simulink model "adcs_sim"  (R2026a)
settings: Solver=ode4  StopTime=t_end  FixedStep=dt
values from neighbouring files (symbols this model uses):
  ephem_moon = [ephem_raw.moon_x, ephem_raw.moon_y, ephem_raw.moon_z]    [init_adcs_params.m]
  ephem_sun = [ephem_raw.sun_x,  ephem_raw.sun_y,  ephem_raw.sun_z]    [init_adcs_params.m]
  ephem_t_sec = seconds(ephem_dt - ephem_epoch)    [init_adcs_params.m]
  epoch_jd = 2461083.5    [init_adcs_params.m]
  h_W0 = [0; 0; 0; 0]    [init_adcs_params.m]
  J = diag([Jx, Jy, Jz])    [Simulator.m]    (also in init_adcs_params.m = diag((mass_sc / 12) * [      sc_dim_y^2 + sc_dim_z^2,      s; summarize_adcs_simulation.m = evalin('base', 'J'))
  omega0 = [0.01; 0.02; 0.0]    [Simulator.m]    (also in init_adcs_params.m = [0.01; -0.005; 0.02]; summarize_adcs_simulation.m = evalin('base', 'omega0'))
  q0 = [1; 0; 0; 0]    [init_adcs_params.m]    (also in launch_adcs_gui.m = q0 / q_norm; summarize_adcs_simulation.m = normalize_quaternion(evalin('base', 'q0')))
settings Model: Creator=akshu  LastModifiedBy=akshu

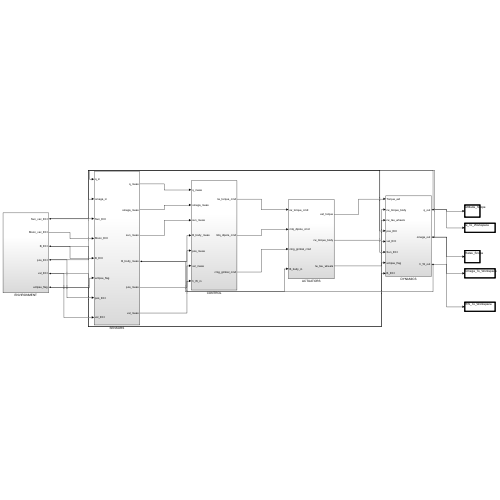
[thumbnail: Simulink's stored preview of the top-level diagram]
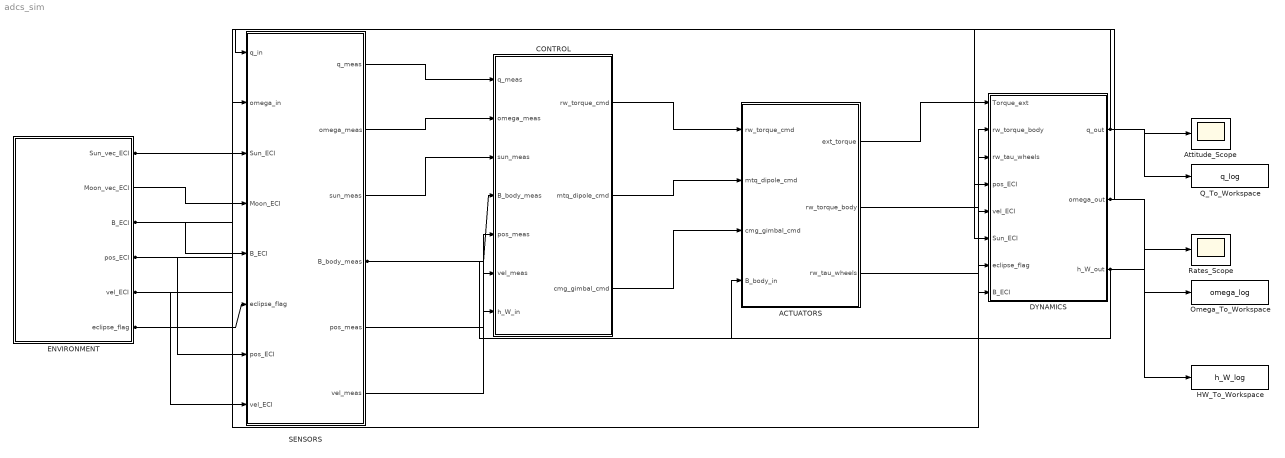
== system adcs_sim ==
  ACTUATORS : Subsystem
  Attitude_Scope : Scope
  CONTROL : Subsystem
  DYNAMICS : Subsystem
  ENVIRONMENT : Subsystem
  HW_To_Workspace : ToWorkspace  VariableName=h_W_log  SaveFormat=Timeseries  SampleTime=-1
  Omega_To_Workspace : ToWorkspace  VariableName=omega_log  SaveFormat=Timeseries  SampleTime=-1
  Q_To_Workspace : ToWorkspace  VariableName=q_log  SaveFormat=Timeseries  SampleTime=-1
  Rates_Scope : Scope
  SENSORS : Subsystem
  wires:
  ENVIRONMENT/1(Sun_vec_ECI) -> SENSORS/3(Sun_ECI), DYNAMICS/6(Sun_ECI)
  ENVIRONMENT/2(Moon_vec_ECI) -> SENSORS/4(Moon_ECI)
  ENVIRONMENT/3(B_ECI) -> SENSORS/5(B_ECI), DYNAMICS/8(B_ECI)
  ENVIRONMENT/4(pos_ECI) -> SENSORS/7(pos_ECI), DYNAMICS/4(pos_ECI)
  ENVIRONMENT/5(vel_ECI) -> SENSORS/8(vel_ECI), DYNAMICS/5(vel_ECI)
  ENVIRONMENT/6(eclipse_flag) -> SENSORS/6(eclipse_flag), DYNAMICS/7(eclipse_flag)
  SENSORS/1(q_meas) -> CONTROL/1(q_meas)
  SENSORS/2(omega_meas) -> CONTROL/2(omega_meas)
  SENSORS/3(sun_meas) -> CONTROL/3(sun_meas)
  SENSORS/4(B_body_meas) -> CONTROL/4(B_body_meas), ACTUATORS/4(B_body_in)
  SENSORS/5(pos_meas) -> CONTROL/5(pos_meas)
  SENSORS/6(vel_meas) -> CONTROL/6(vel_meas)
  DYNAMICS/3(h_W_out) -> CONTROL/7(h_W_in), HW_To_Workspace/1
  CONTROL/1(rw_torque_cmd) -> ACTUATORS/1(rw_torque_cmd)
  CONTROL/2(mtq_dipole_cmd) -> ACTUATORS/2(mtq_dipole_cmd)
  CONTROL/3(cmg_gimbal_cmd) -> ACTUATORS/3(cmg_gimbal_cmd)
  ACTUATORS/1(ext_torque) -> DYNAMICS/1(Torque_ext)
  ACTUATORS/2(rw_torque_body) -> DYNAMICS/2(rw_torque_body)
  ACTUATORS/3(rw_tau_wheels) -> DYNAMICS/3(rw_tau_wheels)
  DYNAMICS/1(q_out) -> SENSORS/1(q_in), Attitude_Scope/1, Q_To_Workspace/1
  DYNAMICS/2(omega_out) -> SENSORS/2(omega_in), Rates_Scope/1, Omega_To_Workspace/1

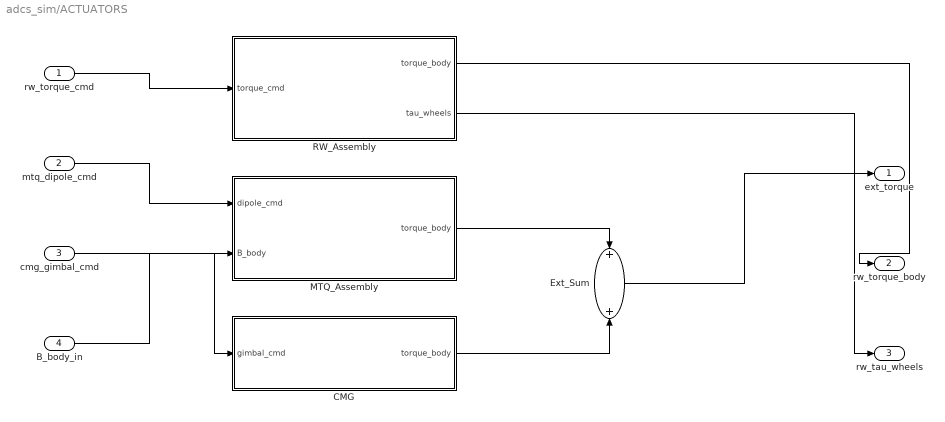
== system adcs_sim/ACTUATORS ==
  rw_torque_cmd : Inport
  mtq_dipole_cmd : Inport  Port=2
  cmg_gimbal_cmd : Inport  Port=3
  B_body_in : Inport  Port=4
  CMG : MATLAB Function  TreatAsAtomicUnit=on
  Ext_Sum : Sum
  MTQ_Assembly : MATLAB Function  TreatAsAtomicUnit=on
  RW_Assembly : MATLAB Function  TreatAsAtomicUnit=on
  ext_torque : Outport
  rw_torque_body : Outport  Port=2
  rw_tau_wheels : Outport  Port=3
  wires:
  rw_torque_cmd/1 -> RW_Assembly/1(torque_cmd)
  mtq_dipole_cmd/1 -> MTQ_Assembly/1(dipole_cmd)
  B_body_in/1 -> MTQ_Assembly/2(B_body)
  cmg_gimbal_cmd/1 -> CMG/1(gimbal_cmd)
  MTQ_Assembly/1(torque_body) -> Ext_Sum/1
  CMG/1(torque_body) -> Ext_Sum/2
  Ext_Sum/1 -> ext_torque/1
  RW_Assembly/1(torque_body) -> rw_torque_body/1
  RW_Assembly/2(tau_wheels) -> rw_tau_wheels/1

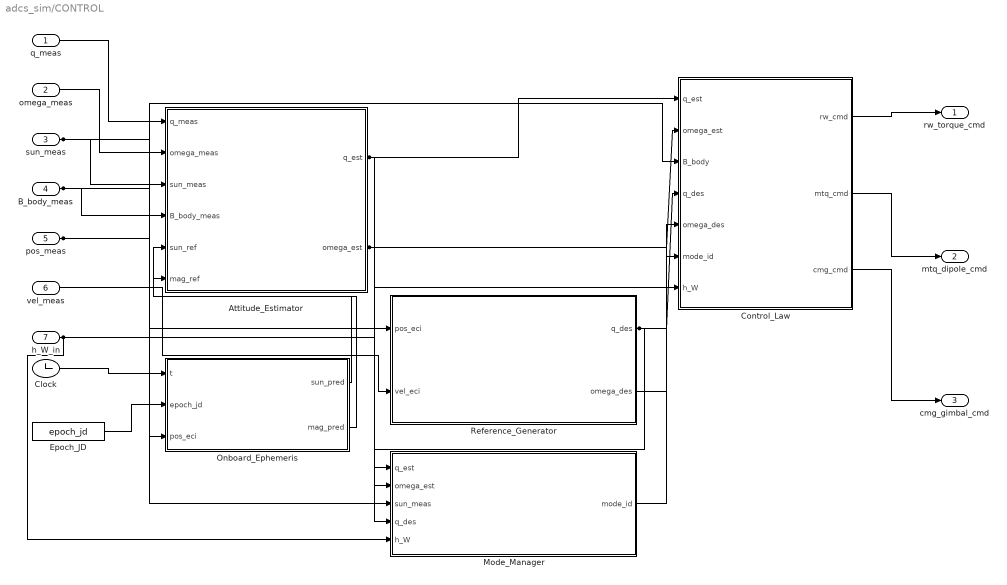
== system adcs_sim/CONTROL ==
  q_meas : Inport
  omega_meas : Inport  Port=2
  sun_meas : Inport  Port=3
  B_body_meas : Inport  Port=4
  pos_meas : Inport  Port=5
  vel_meas : Inport  Port=6
  h_W_in : Inport  Port=7
  Attitude_Estimator : MATLAB Function  TreatAsAtomicUnit=on
  Clock : Clock
  Control_Law : MATLAB Function  TreatAsAtomicUnit=on
  Epoch_JD : Constant  Value=epoch_jd
  Mode_Manager : MATLAB Function  TreatAsAtomicUnit=on
  Onboard_Ephemeris : MATLAB Function  TreatAsAtomicUnit=on
  Reference_Generator : MATLAB Function  TreatAsAtomicUnit=on
  rw_torque_cmd : Outport
  mtq_dipole_cmd : Outport  Port=2
  cmg_gimbal_cmd : Outport  Port=3
  wires:
  Clock/1 -> Onboard_Ephemeris/1(t)
  Epoch_JD/1 -> Onboard_Ephemeris/2(epoch_jd)
  pos_meas/1 -> Onboard_Ephemeris/3(pos_eci), Reference_Generator/1(pos_eci)
  q_meas/1 -> Attitude_Estimator/1(q_meas)
  omega_meas/1 -> Attitude_Estimator/2(omega_meas)
  sun_meas/1 -> Attitude_Estimator/3(sun_meas), Mode_Manager/3(sun_meas)
  B_body_meas/1 -> Attitude_Estimator/4(B_body_meas), Control_Law/3(B_body)
  Onboard_Ephemeris/1(sun_pred) -> Attitude_Estimator/5(sun_ref)
  Onboard_Ephemeris/2(mag_pred) -> Attitude_Estimator/6(mag_ref)
  Attitude_Estimator/1(q_est) -> Control_Law/1(q_est), Mode_Manager/1(q_est)
  Attitude_Estimator/2(omega_est) -> Control_Law/2(omega_est), Mode_Manager/2(omega_est)
  vel_meas/1 -> Reference_Generator/2(vel_eci)
  Reference_Generator/1(q_des) -> Control_Law/4(q_des), Mode_Manager/4(q_des)
  Reference_Generator/2(omega_des) -> Control_Law/5(omega_des)
  h_W_in/1 -> Mode_Manager/5(h_W), Control_Law/7(h_W)
  Mode_Manager/1(mode_id) -> Control_Law/6(mode_id)
  Control_Law/1(rw_cmd) -> rw_torque_cmd/1
  Control_Law/2(mtq_cmd) -> mtq_dipole_cmd/1
  Control_Law/3(cmg_cmd) -> cmg_gimbal_cmd/1

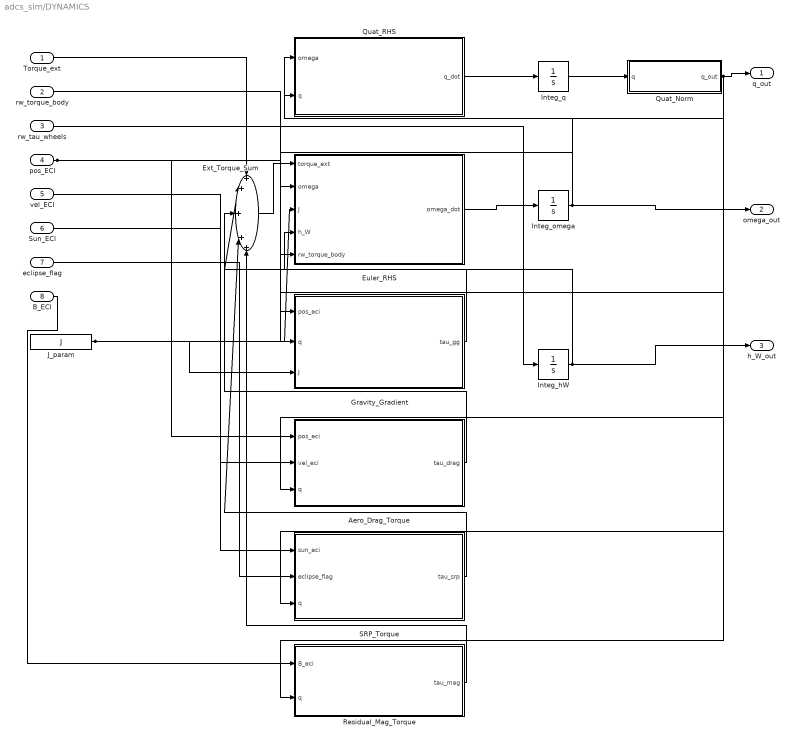
== system adcs_sim/DYNAMICS ==
  Torque_ext : Inport
  rw_torque_body : Inport  Port=2
  rw_tau_wheels : Inport  Port=3
  pos_ECI : Inport  Port=4
  vel_ECI : Inport  Port=5
  Sun_ECI : Inport  Port=6
  eclipse_flag : Inport  Port=7
  B_ECI : Inport  Port=8
  Aero_Drag_Torque : MATLAB Function  TreatAsAtomicUnit=on
  Euler_RHS : MATLAB Function  TreatAsAtomicUnit=on
  Ext_Torque_Sum : Sum  Inputs=+++++
  Gravity_Gradient : MATLAB Function  TreatAsAtomicUnit=on
  Integ_hW : Integrator  InitialCondition=h_W0
  Integ_omega : Integrator  InitialCondition=omega0
  Integ_q : Integrator  InitialCondition=q0
  J_param : Constant  Value=J
  Quat_Norm : MATLAB Function  TreatAsAtomicUnit=on
  Quat_RHS : MATLAB Function  TreatAsAtomicUnit=on
  Residual_Mag_Torque : MATLAB Function  TreatAsAtomicUnit=on
  SRP_Torque : MATLAB Function  TreatAsAtomicUnit=on
  q_out : Outport
  omega_out : Outport  Port=2
  h_W_out : Outport  Port=3
  wires:
  Torque_ext/1 -> Ext_Torque_Sum/1
  Gravity_Gradient/1(tau_gg) -> Ext_Torque_Sum/2
  Aero_Drag_Torque/1(tau_drag) -> Ext_Torque_Sum/3
  SRP_Torque/1(tau_srp) -> Ext_Torque_Sum/4
  Residual_Mag_Torque/1(tau_mag) -> Ext_Torque_Sum/5
  Ext_Torque_Sum/1 -> Euler_RHS/1(torque_ext)
  Integ_omega/1 -> Euler_RHS/2(omega), omega_out/1, Quat_RHS/1(omega)
  J_param/1 -> Euler_RHS/3(J), Gravity_Gradient/3(J)
  Integ_hW/1 -> Euler_RHS/4(h_W), h_W_out/1
  rw_torque_body/1 -> Euler_RHS/5(rw_torque_body)
  Euler_RHS/1(omega_dot) -> Integ_omega/1
  rw_tau_wheels/1 -> Integ_hW/1
  Quat_Norm/1(q_out) -> Quat_RHS/2(q), q_out/1, Gravity_Gradient/2(q), Aero_Drag_Torque/3(q), SRP_Torque/3(q), Residual_Mag_Torque/2(q)
  Quat_RHS/1(q_dot) -> Integ_q/1
  Integ_q/1 -> Quat_Norm/1(q)
  pos_ECI/1 -> Gravity_Gradient/1(pos_eci), Aero_Drag_Torque/1(pos_eci)
  vel_ECI/1 -> Aero_Drag_Torque/2(vel_eci)
  Sun_ECI/1 -> SRP_Torque/1(sun_eci)
  eclipse_flag/1 -> SRP_Torque/2(eclipse_flag)
  B_ECI/1 -> Residual_Mag_Torque/1(B_eci)

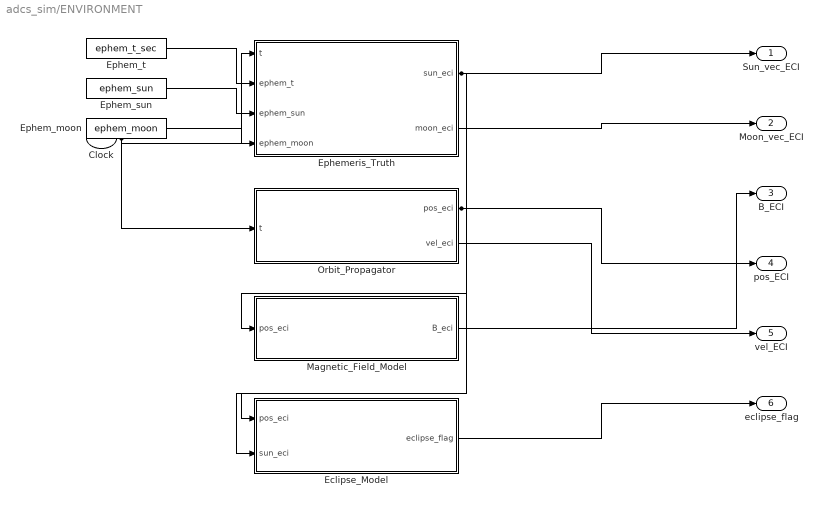
== system adcs_sim/ENVIRONMENT ==
  Clock : Clock
  Eclipse_Model : MATLAB Function  TreatAsAtomicUnit=on
  Ephem_moon : Constant  Value=ephem_moon
  Ephem_sun : Constant  Value=ephem_sun
  Ephem_t : Constant  Value=ephem_t_sec
  Ephemeris_Truth : MATLAB Function  TreatAsAtomicUnit=on
  Magnetic_Field_Model : MATLAB Function  TreatAsAtomicUnit=on
  Orbit_Propagator : MATLAB Function  TreatAsAtomicUnit=on
  Sun_vec_ECI : Outport
  Moon_vec_ECI : Outport  Port=2
  B_ECI : Outport  Port=3
  pos_ECI : Outport  Port=4
  vel_ECI : Outport  Port=5
  eclipse_flag : Outport  Port=6
  wires:
  Clock/1 -> Ephemeris_Truth/1(t), Orbit_Propagator/1(t)
  Ephem_t/1 -> Ephemeris_Truth/2(ephem_t)
  Ephem_sun/1 -> Ephemeris_Truth/3(ephem_sun)
  Ephem_moon/1 -> Ephemeris_Truth/4(ephem_moon)
  Ephemeris_Truth/1(sun_eci) -> Sun_vec_ECI/1, Eclipse_Model/2(sun_eci)
  Ephemeris_Truth/2(moon_eci) -> Moon_vec_ECI/1
  Orbit_Propagator/1(pos_eci) -> pos_ECI/1, Magnetic_Field_Model/1(pos_eci), Eclipse_Model/1(pos_eci)
  Orbit_Propagator/2(vel_eci) -> vel_ECI/1
  Magnetic_Field_Model/1(B_eci) -> B_ECI/1
  Eclipse_Model/1(eclipse_flag) -> eclipse_flag/1

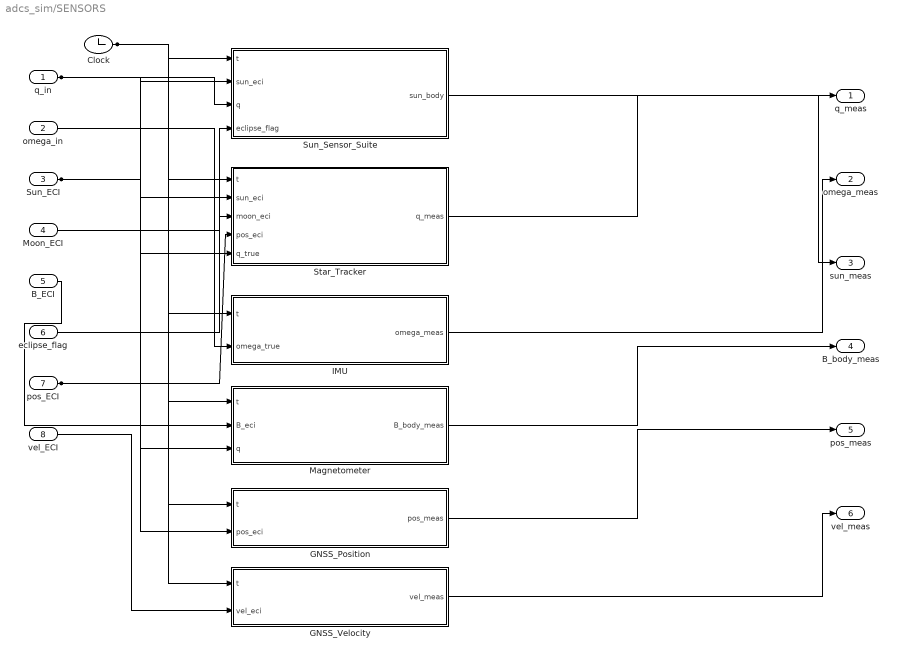
== system adcs_sim/SENSORS ==
  q_in : Inport
  omega_in : Inport  Port=2
  Sun_ECI : Inport  Port=3
  Moon_ECI : Inport  Port=4
  B_ECI : Inport  Port=5
  eclipse_flag : Inport  Port=6
  pos_ECI : Inport  Port=7
  vel_ECI : Inport  Port=8
  Clock : Clock
  GNSS_Position : MATLAB Function  TreatAsAtomicUnit=on
  GNSS_Velocity : MATLAB Function  TreatAsAtomicUnit=on
  IMU : MATLAB Function  TreatAsAtomicUnit=on
  Magnetometer : MATLAB Function  TreatAsAtomicUnit=on
  Star_Tracker : MATLAB Function  TreatAsAtomicUnit=on
  Sun_Sensor_Suite : MATLAB Function  TreatAsAtomicUnit=on
  q_meas : Outport
  omega_meas : Outport  Port=2
  sun_meas : Outport  Port=3
  B_body_meas : Outport  Port=4
  pos_meas : Outport  Port=5
  vel_meas : Outport  Port=6
  wires:
  Clock/1 -> Sun_Sensor_Suite/1(t), Star_Tracker/1(t), IMU/1(t), Magnetometer/1(t), GNSS_Position/1(t), GNSS_Velocity/1(t)
  Sun_ECI/1 -> Sun_Sensor_Suite/2(sun_eci), Star_Tracker/2(sun_eci)
  q_in/1 -> Sun_Sensor_Suite/3(q), Star_Tracker/5(q_true), Magnetometer/3(q)
  eclipse_flag/1 -> Sun_Sensor_Suite/4(eclipse_flag)
  Moon_ECI/1 -> Star_Tracker/3(moon_eci)
  pos_ECI/1 -> Star_Tracker/4(pos_eci), GNSS_Position/2(pos_eci)
  omega_in/1 -> IMU/2(omega_true)
  B_ECI/1 -> Magnetometer/2(B_eci)
  vel_ECI/1 -> GNSS_Velocity/2(vel_eci)
  Star_Tracker/1(q_meas) -> q_meas/1
  IMU/1(omega_meas) -> omega_meas/1
  Sun_Sensor_Suite/1(sun_body) -> sun_meas/1
  Magnetometer/1(B_body_meas) -> B_body_meas/1
  GNSS_Position/1(pos_meas) -> pos_meas/1
  GNSS_Velocity/1(vel_meas) -> vel_meas/1

== matlab function adcs_sim/CONTROL/Onboard_Ephemeris ==
  data: t input double size=1; sun_pred output double size=[3 1]; epoch_jd input double size=1; pos_eci input double size=[3 1]; mag_pred output double size=[3 1]
function [sun_pred, mag_pred] = fcn(t, epoch_jd, pos_eci)
%#codegen
% Deterministic reference vectors used during compile hardening.
  sun_pred = [1; 0; 0];
  mag_pred = [0; 0; 1];
end

== matlab function adcs_sim/CONTROL/Attitude_Estimator ==
  data: q_meas input double size=[4 1]; q_est output double size=[4 1]; omega_meas input double size=[3 1]; sun_meas input double size=[3 1]; B_body_meas input double size=[3 1]; sun_ref input double size=[3 1]; mag_ref input double size=[3 1]; omega_est output double size=[3 1]
function [q_est, omega_est] = fcn(q_meas, omega_meas, sun_meas, B_body_meas, sun_ref, mag_ref)
%#codegen
% Compile-stable estimator passthrough.
  qn = sqrt(q_meas(1)^2 + q_meas(2)^2 + q_meas(3)^2 + q_meas(4)^2);
  if qn > 1e-12
      q_est = q_meas / qn;
  else
      q_est = [1; 0; 0; 0];
  end
  if q_est(1) < 0
      q_est = -q_est;
  end
  omega_est = omega_meas;
end

== matlab function adcs_sim/CONTROL/Reference_Generator ==
  data: pos_eci input double size=[3 1]; q_des output double size=[4 1]; vel_eci input double size=[3 1]; omega_des output double size=[3 1]
function [q_des, omega_des] = fcn(pos_eci, vel_eci)
%#codegen
% Compile-stable identity reference.
  q_des = [1; 0; 0; 0];
  omega_des = [0; 0; 0];
end

== matlab function adcs_sim/CONTROL/Mode_Manager ==
  data: q_est input double size=[4 1]; mode_id output double size=1; omega_est input double size=[3 1]; sun_meas input double size=[3 1]; q_des input double size=[4 1]; h_W input double size=[4 1]
function mode_id = fcn(q_est, omega_est, sun_meas, q_des, h_W)
%#codegen
% Compile-stable constant mode selection.
  mode_id = 2;
end

== matlab function adcs_sim/CONTROL/Control_Law ==
  data: q_est input double size=[4 1]; rw_cmd output double size=[3 1]; omega_est input double size=[3 1]; B_body input double size=[3 1]; q_des input double size=[4 1]; omega_des input double size=[3 1]; mode_id input double size=1; h_W input double size=[4 1]; mtq_cmd output double size=[3 1]; cmg_cmd output double size=[3 1]
function [rw_cmd, mtq_cmd, cmg_cmd] = fcn(q_est, omega_est, B_body, q_des, omega_des, mode_id, h_W)
%#codegen
% Compile-stable zero-torque fallback.
  rw_cmd = [0; 0; 0];
  mtq_cmd = [0; 0; 0];
  cmg_cmd = [0; 0; 0];
end

== matlab function adcs_sim/ENVIRONMENT/Orbit_Propagator ==
  data: t input double size=1; pos_eci output double size=[3 1]; vel_eci output double size=[3 1]
function [pos_eci, vel_eci] = fcn(t)
%#codegen
% Compile-stable fixed LEO state fallback.
  pos_eci = [6871000; 0; 0];
  vel_eci = [0; 7616.5; 0];
end

== matlab function adcs_sim/ACTUATORS/RW_Assembly ==
  data: torque_cmd input double size=[3 1]; torque_body output double size=[3 1]; tau_wheels output double size=[4 1]
function [torque_body, tau_wheels] = fcn(torque_cmd)
%#codegen
% Compile-stable zero-torque fallback.
  torque_body = [0; 0; 0];
  tau_wheels = [0; 0; 0; 0];
end

== matlab function adcs_sim/ACTUATORS/MTQ_Assembly ==
  data: dipole_cmd input double size=[3 1]; torque_body output double size=[3 1]; B_body input double size=[3 1]
function torque_body = fcn(dipole_cmd, B_body)
%#codegen
% Compile-stable zero-torque fallback.
  torque_body = [0; 0; 0];
end

== matlab function adcs_sim/ACTUATORS/CMG ==
  data: gimbal_cmd input double size=[3 1]; torque_body output double size=[3 1]
function torque_body = fcn(gimbal_cmd)
%#codegen
% Compile-stable zero-torque fallback.
  torque_body = [0; 0; 0];
end

== matlab function adcs_sim/DYNAMICS/Euler_RHS ==
  data: torque_ext input double size=[3 1]; omega_dot output double size=[3 1]; omega input double size=[3 1]; J input double size=[3 3]; h_W input double size=[4 1]; rw_torque_body input double size=[3 1]
function omega_dot = fcn(torque_ext, omega, J, h_W, rw_torque_body)
%#codegen
% Euler equation with reaction-wheel momentum coupling:
%   omega_dot = J \ (torque_ext - omega×(J*omega + A_W*h_W) - rw_torque_body)

  beta = atan(1/sqrt(2));
  cb = cos(beta); sb = sin(beta);
  A_W = [ cb,  0, -cb,  0;
           0, cb,   0, -cb;
          sb, sb,  sb,  sb ];

  H_total = J * omega + A_W * h_W;
  cross_term = [ omega(2)*H_total(3) - omega(3)*H_total(2);
                 omega(3)*H_total(1) - omega(1)*H_total(3);
                 omega(1)*H_total(2) - omega(2)*H_total(1) ];
  omega_dot = J \ (torque_ext - cross_term - rw_torque_body);
end

== matlab function adcs_sim/DYNAMICS/Gravity_Gradient ==
  data: pos_eci input double size=[3 1]; tau_gg output double size=[3 1]; q input double size=[4 1]; J input double size=[3 3]
function tau_gg = fcn(pos_eci, q, J)
%#codegen
% Gravity-gradient torque in body frame.
% tau_gg = (3*mu/R^3) * cross(r_body, J*r_body)

  mu = 3.986004418e14;
  R = sqrt(pos_eci(1)^2 + pos_eci(2)^2 + pos_eci(3)^2);
  if R < 1e-9
      tau_gg = [0; 0; 0];
      return;
  end

  r_hat_eci = -pos_eci / R;

  q0 = q(1); q1 = q(2); q2 = q(3); q3 = q(4);
  % Use the same ECI->body DCM convention as the active sensor models.
  C_bi = [1-2*(q2*q2+q3*q3),   2*(q1*q2+q0*q3),   2*(q1*q3-q0*q2);
            2*(q1*q2-q0*q3), 1-2*(q1*q1+q3*q3),   2*(q2*q3+q0*q1);
            2*(q1*q3+q0*q2),   2*(q2*q3-q0*q1), 1-2*(q1*q1+q2*q2)];

  r_body = C_bi * r_hat_eci;
  Jr = J * r_body;
  c = [r_body(2)*Jr(3)-r_body(3)*Jr(2);
       r_body(3)*Jr(1)-r_body(1)*Jr(3);
       r_body(1)*Jr(2)-r_body(2)*Jr(1)];
  tau_gg = (3*mu/(R^3)) * c;
end

== matlab function adcs_sim/DYNAMICS/Aero_Drag_Torque ==
  data: pos_eci input double size=[3 1]; tau_drag output double size=[3 1]; vel_eci input double size=[3 1]; q input double size=[4 1]
function tau_drag = fcn(pos_eci, vel_eci, q)
%#codegen
% Compile-stable zero disturbance fallback.
  tau_drag = [0; 0; 0];
end

== matlab function adcs_sim/DYNAMICS/SRP_Torque ==
  data: sun_eci input double size=[3 1]; tau_srp output double size=[3 1]; eclipse_flag input double size=1; q input double size=[4 1]
function tau_srp = fcn(sun_eci, eclipse_flag, q)
%#codegen
% Compile-stable zero disturbance fallback.
  tau_srp = [0; 0; 0];
end

== matlab function adcs_sim/DYNAMICS/Residual_Mag_Torque ==
  data: B_eci input double size=[3 1]; tau_mag output double size=[3 1]; q input double size=[4 1]
function tau_mag = fcn(B_eci, q)
%#codegen
% Compile-stable zero disturbance fallback.
  tau_mag = [0; 0; 0];
end

== matlab function adcs_sim/ENVIRONMENT/Ephemeris_Truth ==
  data: t input double size=1; sun_eci output double size=[3 1]; ephem_t input; ephem_sun input; ephem_moon input; moon_eci output double size=[3 1]
function [sun_eci, moon_eci] = fcn(t, ephem_t, ephem_sun, ephem_moon)
%#codegen
% Ground-truth Sun & Moon direction vectors interpolated from
% pre-loaded ephemeris CSV data (ephemeris_2026_weekly.csv).
%
% Inputs:  t          – simulation time [s]
%          ephem_t    – [Nx1] time breakpoints [s] from epoch
%          ephem_sun  – [Nx3] Sun unit direction vectors (ECI)
%          ephem_moon – [Nx3] Moon unit direction vectors (ECI)
% Outputs: sun_eci    – Sun direction unit vector ECI [3x1]
%          moon_eci   – Moon direction unit vector ECI [3x1]

  N = size(ephem_t, 1);

  % ── Clamp to data range ──
  tc = t;
  if tc < ephem_t(1)
      tc = ephem_t(1);
  elseif tc > ephem_t(N)
      tc = ephem_t(N);
  end

  % ── Find bracketing interval  (linear search, N is small ~53) ──
  idx = 1;
  for k = 1:N-1
      if ephem_t(k+1) >= tc
          idx = k;
          break;
      end
  end

  % ── Linear interpolation fraction ──
  dt_seg = ephem_t(idx+1) - ephem_t(idx);
  if dt_seg > 0
      frac = (tc - ephem_t(idx)) / dt_seg;
  else
      frac = 0;
  end

  % ── Interpolate Sun ──
  s1 = ephem_sun(idx, :)';
  s2 = ephem_sun(idx+1, :)';
  sun_raw = s1 + frac * (s2 - s1);
  sn = sqrt(sun_raw(1)^2 + sun_raw(2)^2 + sun_raw(3)^2);
  if sn > 0
      sun_eci = sun_raw / sn;
  else
      sun_eci = [1; 0; 0];
  end

  % ── Interpolate Moon ──
  m1 = ephem_moon(idx, :)';
  m2 = ephem_moon(idx+1, :)';
  moon_raw = m1 + frac * (m2 - m1);
  mn = sqrt(moon_raw(1)^2 + moon_raw(2)^2 + moon_raw(3)^2);
  if mn > 0
      moon_eci = moon_raw / mn;
  else
      moon_eci = [0; 1; 0];
  end
end

== matlab function adcs_sim/DYNAMICS/Quat_RHS ==
  data: omega input double size=[3 1]; q_dot output double size=[4 1]; q input double size=[4 1]
function q_dot = fcn(omega, q)
%#codegen
% Quaternion kinematics: q_dot = 0.5 * Omega(omega) * q
% Convention: q = [q0; q1; q2; q3]  (scalar-first)

  wx = omega(1); wy = omega(2); wz = omega(3);

  % Omega matrix for scalar-first convention
  Omega = [  0,  -wx, -wy, -wz;
            wx,    0,  wz, -wy;
            wy, -wz,    0,  wx;
            wz,  wy, -wx,    0 ];

  q_dot = 0.5 * Omega * q;
end

== matlab function adcs_sim/DYNAMICS/Quat_Norm ==
  data: q input double size=[4 1]; q_out output double size=[4 1]
function q_out = fcn(q)
%#codegen
% Normalise quaternion.
  n = sqrt(q(1)^2 + q(2)^2 + q(3)^2 + q(4)^2);
  if n > 0
      q_out = q / n;
  else
      q_out = [1; 0; 0; 0];
  end
end

== matlab function adcs_sim/ENVIRONMENT/Magnetic_Field_Model ==
  data: pos_eci input double size=[3 1]; B_eci output double size=[3 1]
function B_eci = fcn(pos_eci)
%#codegen
% Compile-stable literal magnetic field fallback.
  B_eci = [0; 0; 3.12e-5];
end

== matlab function adcs_sim/ENVIRONMENT/Eclipse_Model ==
  data: pos_eci input double size=[3 1]; eclipse_flag output double size=1; sun_eci input double size=[3 1]
function eclipse_flag = fcn(pos_eci, sun_eci)
%#codegen
% Compile-stable sunlit fallback.
  eclipse_flag = 0.0;
end

== matlab function adcs_sim/SENSORS/Sun_Sensor_Suite ==
  data: t input double size=1; sun_body output double size=[3 1]; sun_eci input double size=[3 1]; q input double size=[4 1]; eclipse_flag input double size=1
function sun_body = fcn(t, sun_eci, q, eclipse_flag)
%#codegen
% Deterministic sun-vector body rotation with eclipse gating.
  if eclipse_flag > 0.5
      sun_body = [0; 0; 0];
      return;
  end

  sun_mag = sqrt(sum(sun_eci.^2));
  if sun_mag < 1e-9
      sun_body = [0; 0; 0];
      return;
  end
  s_hat = sun_eci / sun_mag;

  q0=q(1); q1=q(2); q2=q(3); q3=q(4);
  R = [1-2*(q2^2+q3^2),  2*(q1*q2+q0*q3),  2*(q1*q3-q0*q2);
       2*(q1*q2-q0*q3),  1-2*(q1^2+q3^2),  2*(q2*q3+q0*q1);
       2*(q1*q3+q0*q2),  2*(q2*q3-q0*q1),  1-2*(q1^2+q2^2)];
  sun_body = R * s_hat;
end

== matlab function adcs_sim/SENSORS/Star_Tracker ==
  data: t input double size=1; q_meas output double size=[4 1]; sun_eci input double size=[3 1]; moon_eci input double size=[3 1]; pos_eci input double size=[3 1]; q_true input double size=[4 1]
function q_meas = fcn(t, sun_eci, moon_eci, pos_eci, q_true)
%#codegen
% Deterministic passthrough used during compile hardening.
  q_meas = q_true;
end

== matlab function adcs_sim/SENSORS/IMU ==
  data: t input double size=1; omega_meas output double size=[3 1]; omega_true input double size=[3 1]
function omega_meas = fcn(t, omega_true)
%#codegen
% Temporary passthrough used to isolate MATLAB Function analysis issues.
  omega_meas = omega_true;
end

== matlab function adcs_sim/SENSORS/Magnetometer ==
  data: t input double size=1; B_body_meas output double size=[3 1]; B_eci input double size=[3 1]; q input double size=[4 1]
function B_body_meas = fcn(t, B_eci, q)
%#codegen
% Deterministic body-frame field rotation.
  B_body_meas = zeros(3,1);
  qn = max(sqrt(q(1)^2 + q(2)^2 + q(3)^2 + q(4)^2), 1e-12);
  q0 = q(1) / qn;
  q1 = q(2) / qn;
  q2 = q(3) / qn;
  q3 = q(4) / qn;

  c11 = 1 - 2*(q2*q2 + q3*q3);
  c12 = 2*(q1*q2 + q0*q3);
  c13 = 2*(q1*q3 - q0*q2);
  c21 = 2*(q1*q2 - q0*q3);
  c22 = 1 - 2*(q1*q1 + q3*q3);
  c23 = 2*(q2*q3 + q0*q1);
  c31 = 2*(q1*q3 + q0*q2);
  c32 = 2*(q2*q3 - q0*q1);
  c33 = 1 - 2*(q1*q1 + q2*q2);

  bx = c11*B_eci(1) + c12*B_eci(2) + c13*B_eci(3);
  by = c21*B_eci(1) + c22*B_eci(2) + c23*B_eci(3);
  bz = c31*B_eci(1) + c32*B_eci(2) + c33*B_eci(3);

  B_body_meas(1) = bx;
  B_body_meas(2) = by;
  B_body_meas(3) = bz;
end

== matlab function adcs_sim/SENSORS/GNSS_Position ==
  data: t input double size=1; pos_meas output double size=[3 1]; pos_eci input double size=[3 1]
function pos_meas = fcn(t, pos_eci)
%#codegen
% Temporary passthrough used to isolate MATLAB Function analysis issues.
  pos_meas = pos_eci;
end

== matlab function adcs_sim/SENSORS/GNSS_Velocity ==
  data: t input double size=1; vel_meas output double size=[3 1]; vel_eci input double size=[3 1]
function vel_meas = fcn(t, vel_eci)
%#codegen
% Temporary passthrough used to isolate MATLAB Function analysis issues.
  vel_meas = vel_eci;
end
